simulink model "intersampling_ol"  (R2023a)
settings: Solver=VariableStepAuto  StartTime=0.0  StopTime=10.0  RelTol=1e-3
settings Model: Creator=isaac  LastModifiedBy=isaac

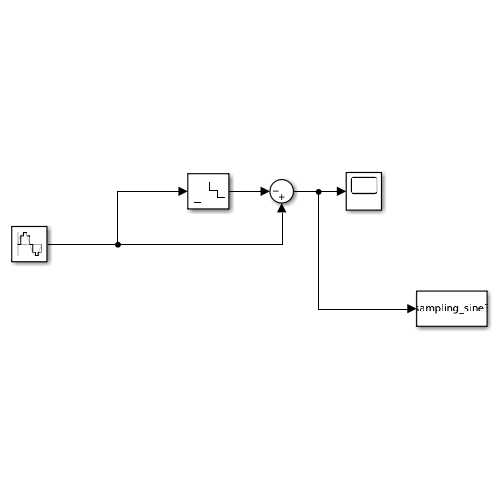
[thumbnail: Simulink's stored preview of the top-level diagram]
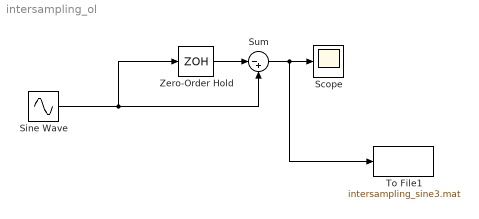
== system intersampling_ol ==
  Scope : Scope
  Sine Wave : Sin  Frequency=80*pi  SampleTime=1/4000
  Sum : Sum  Inputs=|-+
  To File1 : ToFile  Filename=intersampling_sine3.mat  MatrixName=data  SampleTime=1/4000
  Zero-Order Hold : ZeroOrderHold  SampleTime=1/1234
  wires:
  Zero-Order Hold/1 -> Sum/1
  Sine Wave/1 -> Sum/2, Zero-Order Hold/1
  Sum/1 -> To File1/1, Scope/1
